simulink model "NodeMCU_Simulink_LED"  (R2024a)
settings: Solver=VariableStepAuto  StartTime=0.0  StopTime=10.0  RelTol=1e-3
libraries: arduinolib x1
settings Model: SimulationMode=external  Creator=ammaa  LastModifiedBy=ammaa
settings GRTTargetCC: ExtMode=on  ExtModeTransport=1  ExtModeMexFile=ext_serial_win32_comm

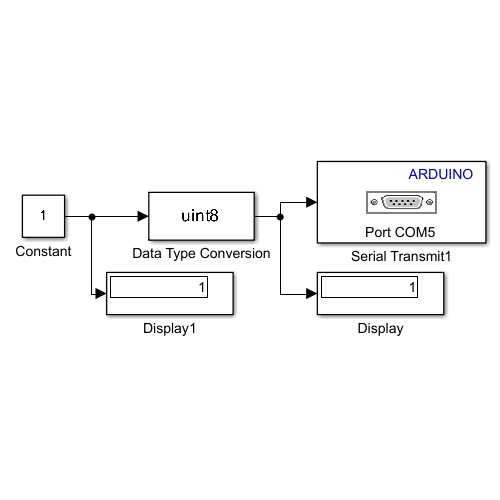
[thumbnail: Simulink's stored preview of the top-level diagram]
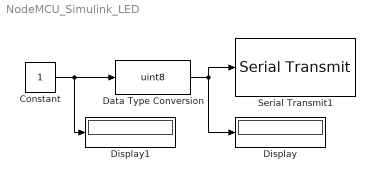
== system NodeMCU_Simulink_LED ==
  Constant : Constant
  Data Type Conversion : DataTypeConversion  OutDataTypeStr=uint8  SaturateOnIntegerOverflow=off  RndMeth=Floor
  Display : Display
  Display1 : Display
  Serial Transmit1 : arduinolib/Serial Transmit  portNumber=COM5  sendmode=write  sendformat=Decimal  floatprecision=2  header=[]  terminator=[]  blockPlatform=arduino
  wires:
  Constant/1 -> Display1/1, Data Type Conversion/1
  Data Type Conversion/1 -> Display/1, Serial Transmit1/1
